simulink model "fxpdemo_lead_lag"  (Simulink 7.6)
settings: Solver=FixedStepDiscrete  SolverMode=SingleTasking  StartTime=0.0  StopTime=7.95  FixedStep=SampleTime  RelTol=1e-3  AbsTol=1e-6
PreLoadFcn:
  | preload_lead_lag
values from neighbouring files (symbols this model uses):
  SampleTime = 0.01    [preload_state_space.m]
undefined symbols (not defined in the file or in its folder): LagKdc, LagZeroZ, LeadKdc, LeadZeroZ, PoleZ
libraries: simulink x2
Description:
  | Fixed-Point Lead and Lag Filters
  | 
  | Sample fixed-point implementations of a discrete lead filter and a discrete lag filter
  | along with reference implementations in floating point.
CloseFcn:
  | close_lead_lag
settings Model: MinMaxOverflowLogging=MinMaxAndOverflow  Creator=The MathWorks Inc.  CovMetricSettings=d  ExtModeTrigMode=oneshot  ExtModeArmWhenConnect=off  ExtModeAutoUpdateStatusClock=off
settings DataIOCC: LimitDataPoints=off  SignalLoggingName=sigsOut
settings OptimizationCC: BooleanDataType=off  InitFltsAndDblsToZero=on  EfficientMapNaN2IntZero=off
settings DebuggingCC: SaveWithParameterizedLinksMsg=none  SignalResolutionControl=TryResolveAllWithWarning  SolverPrmCheckMsg=none  MultiTaskDSMMsg=warning  MultiTaskCondExecSysMsg=none  SigSpecEnsureSampleTimeMsg=none  IntegerOverflowMsg=none  ParameterDowncastMsg=warning  ParameterOverflowMsg=warning  ParameterPrecisionLossMsg=none  StrictBusMsg=None
settings HardwareCC: TargetUnknown=on
settings RTWCC: IncludeERTFirstTime=on
settings GRTTargetCC: TargetFcnLib=ansi_tfl_tmw.mat

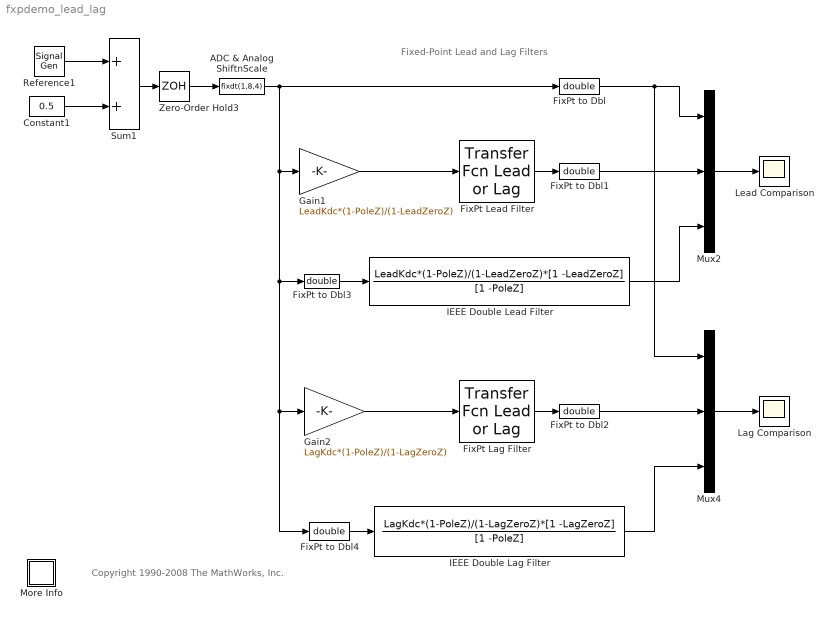
== system fxpdemo_lead_lag ==
  note: Fixed-Point Lead and Lag Filters
  note: Copyright 1990-2008 The MathWorks, Inc.
  ADC & Analog ShiftnScale : DataTypeConversion  OutDataTypeStr=fixdt(1,8,4)  RndMeth=Nearest  SaturateOnIntegerOverflow=on
  Constant1 : Constant  Value=0.5
  FixPt Lag Filter : simulink/Discrete/Transfer Fcn Lead or Lag  SystemSampleTime=-1  PoleZ=PoleZ  ZeroZ=LagZeroZ  ICPrevOutput=0.0  ICPrevInput=0.0  DoSatur=off
  FixPt Lead Filter : simulink/Discrete/Transfer Fcn Lead or Lag  SystemSampleTime=-1  PoleZ=PoleZ  ZeroZ=LeadZeroZ  ICPrevOutput=0.0  ICPrevInput=0.0  DoSatur=off
  FixPt to Dbl{,1..4} (5 alike) : DataTypeConversion  OutDataTypeStr=double
  Gain1 : Gain  Gain=LeadKdc*(1-PoleZ)/(1-LeadZeroZ)
  Gain2 : Gain  Gain=LagKdc*(1-PoleZ)/(1-LagZeroZ)
  IEEE Double Lag Filter : DiscreteFilter  Numerator=LagKdc*(1-PoleZ)/(1-LagZeroZ)*[1 -LagZeroZ]  Denominator=[1 -PoleZ]  SampleTime=SampleTime
  IEEE Double Lead Filter : DiscreteFilter  Numerator=LeadKdc*(1-PoleZ)/(1-LeadZeroZ)*[1 -LeadZeroZ]  Denominator=[1 -PoleZ]  SampleTime=SampleTime
  Lag Comparison : Scope
      settings: TickLabels=on  YMin=-3  YMax=4  SaveName=LagCompare
  Lead Comparison : Scope
      settings: TickLabels=on  TimeRange=8  YMin=-3  YMax=3  SaveName=LeadCompare
  More Info : Subsystem
      settings: OpenFcn=showdemo(bdroot(gcs))
      mask Display: disp('?')
  Mux2 : Mux  Inputs=3
  Mux4 : Mux  Inputs=3
  Reference1 : SignalGenerator  WaveForm=square  Amplitude=-1.5  Frequency=1/8
  Sum1 : Sum  Inputs=2  SaturateOnIntegerOverflow=on  InputSameDT=on  OutDataTypeStr=Inherit: Same as first input
  Zero-Order Hold3 : ZeroOrderHold  SampleTime=SampleTime
  wires:
  Reference1/1 -> Sum1/1
  Constant1/1 -> Sum1/2
  Zero-Order Hold3/1 -> ADC & Analog ShiftnScale/1
  Sum1/1 -> Zero-Order Hold3/1
  ADC & Analog ShiftnScale/1 -> FixPt to Dbl/1, Gain1/1, FixPt to Dbl3/1, FixPt to Dbl4/1, Gain2/1
  FixPt to Dbl/1 -> Mux2/1, Mux4/1
  FixPt to Dbl1/1 -> Mux2/2
  IEEE Double Lead Filter/1 -> Mux2/3
  FixPt Lag Filter/1 -> FixPt to Dbl2/1
  IEEE Double Lag Filter/1 -> Mux4/3
  FixPt to Dbl4/1 -> IEEE Double Lag Filter/1
  FixPt to Dbl3/1 -> IEEE Double Lead Filter/1
  FixPt to Dbl2/1 -> Mux4/2
  Mux2/1 -> Lead Comparison/1
  Mux4/1 -> Lag Comparison/1
  FixPt Lead Filter/1 -> FixPt to Dbl1/1
  Gain1/1 -> FixPt Lead Filter/1
  Gain2/1 -> FixPt Lag Filter/1

== system fxpdemo_lead_lag/More Info ==
